simulink model "blockdemo"  (Simulink 6.3)
settings: Solver=FixedStepDiscrete  StartTime=0.0  StopTime=20.0  RelTol=1e-3
InitFcn:
  | %% DSPBuilder Start
  | alt_dspbuilder_update_model(bdroot)
  | %% DSPBuilder End
libraries: allblocks_alteradspbuilder2 x10
settings Model: Creator=cpurcell  LastModifiedBy=delphick
settings DebuggingCC: MultiTaskDSMMsg=error

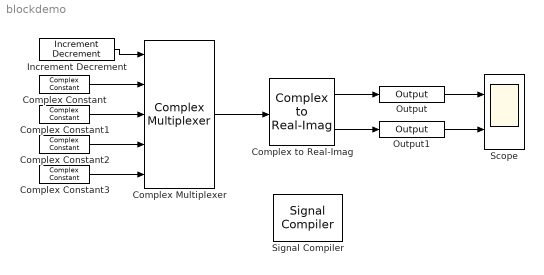
== system blockdemo ==
  Complex Constant : allblocks_alteradspbuilder2/Complex Constant  mask_cst_real=2  mask_cst_imag=4  BusType=Signed Integer  bwl=8  bwr=0  SpecifyClock=off
  Complex Constant1 : allblocks_alteradspbuilder2/Complex Constant  mask_cst_real=4  mask_cst_imag=8  BusType=Signed Integer  bwl=8  bwr=0  SpecifyClock=off
  Complex Constant2 : allblocks_alteradspbuilder2/Complex Constant  mask_cst_real=7  mask_cst_imag=19  BusType=Signed Integer  bwl=8  bwr=0  SpecifyClock=off
  Complex Constant3 : allblocks_alteradspbuilder2/Complex Constant  mask_cst_real=11  mask_cst_imag=23  BusType=Signed Integer  bwl=8  bwr=0  SpecifyClock=off
  Complex Multiplexer : allblocks_alteradspbuilder2/Complex Multiplexer  numInputs=4  pipeline=1  oneHot=off  use_ena=off  use_aclr=off
  Complex to Real-Imag : allblocks_alteradspbuilder2/Complex to Real-Imag  BusType=Signed Integer  bwl=10  bwr=0
  Increment Decrement : allblocks_alteradspbuilder2/Increment Decrement  BusType=Signed Integer  bwl=2  bwr=8  SpecifyClock=off  clr_value=0  direction=Increment  phase_selection=1  use_ena=off  use_sclr=off
  Output : allblocks_alteradspbuilder2/Output  iofile=C:\workspace_clean\Documentation\DesignExamples\Tutorials\UnitBlocks\Complex\ComplexMultiplexer\tb_blockdemo\blockdemo_Output.capture  BusType=Inferred  bwl=8  bwr=0  PORTTYPE=Output
  Output1 : allblocks_alteradspbuilder2/Output  iofile=C:\workspace_clean\Documentation\DesignExamples\Tutorials\UnitBlocks\Complex\ComplexMultiplexer\tb_blockdemo\blockdemo_Output1.capture  BusType=Inferred  bwl=8  bwr=0  PORTTYPE=Output
  Scope : Scope  NumInputPorts=2
      settings: TimeRange=20  YMin=-1~-1  YMax=12~25
  Signal Compiler : allblocks_alteradspbuilder2/Signal Compiler  DeviceFamily=Stratix IV  DeviceName=AUTO  EnableSignalTap=off  SignalTapDepth=128  UseBoardBlock=off  StpUseDefaultClock=on  StpClock=clock
  wires:
  Complex Constant/1 -> Complex Multiplexer/2
  Complex Constant1/1 -> Complex Multiplexer/3
  Complex Constant2/1 -> Complex Multiplexer/4
  Complex Constant3/1 -> Complex Multiplexer/5
  Complex Multiplexer/1 -> Complex to Real-Imag/1
  Complex to Real-Imag/1 -> Output/1
  Complex to Real-Imag/2 -> Output1/1
  Output/1 -> Scope/1
  Output1/1 -> Scope/2
  Increment Decrement/1 -> Complex Multiplexer/1
